simulink subsystem "In_Plane_ModelArchitecture"  (R2025b)
settings: Solver=VariableStepAuto  StartTime=0.0  StopTime=10.0  RelTol=1e-3
undefined symbols (not defined in the file or in its folder): AeroLiftCff, AeroLongDrgCff, AeroMotoEffctArea, AeroPitchMomentCff, AeroPitchMomentLngth, AeroRltWindAngVect, AeroSideFrcCff, AeroYawMomentCff, aMode, BrkFrntBrkActrBore, BrkFrntBrkActrPrsBpt, BrkFrntBrkPadMeanRadius, BrkFrntBrkTrqTbl, BrkFrntIntrnRadius, BrkFrntKinFricCff, BrkFrntPadNum, BrkFrntShoePinToDrumCntrDst, BrkFrntShoePinToFrcAppDst, BrkFrntShoePinToPadEndAng, BrkFrntShoePinToPadStartAng, BrkFrntStcFricCff, BrkFrntWhlSpdBpt, BrkRearBrkActrBore, BrkRearBrkActrPrsBpt, BrkRearBrkPadMeanRadius, BrkRearBrkTrqTbl, BrkRearIntrnRadius, BrkRearKinFricCff, BrkRearPadNum, BrkRearShoePinToDrumCntrDst, BrkRearShoePinToFrcAppDst, BrkRearShoePinToPadEndAng, BrkRearShoePinToPadStartAng, BrkRearStcFricCff, BrkRearWhlSpdBpt, EnvAbsPrs, EnvAirTemp, FrkFrL0, FrmAng0, g, GasCnst, InitFrkLngth, InitMainFrmPitchAng, InitRearArmPitchAng, InitRearCntctPtchLatVel, InitRearCntctPtchLongVel, InitRearCntctPtchY, InitRearCntctPtchZ, InitRollAng, InitYawAng, MotoFrmLngth, MotoFrmMass, MotoGrvty, MotoLatOfst, MotoLongOfst, MotoLowrFrntFrkMass, MotoPtchOfst, MotoRearArmLngth, MotoRearArmMass, MotoRollOfst ... (+25)
libraries: sm_lib x309, nesl_utility_internal x158, nesl_utility x7, autolibsharedcoupling x6, vehdynlibtire x6, sharedtransform x4, shared6dof x1, matrix_library x1, vehdynlibeomcommon x1
(part 5 of 10)

== system In_Plane_ModelArchitecture/Chassis, Tires, and Areo/Chassis Body, Suspension, and Steering/CHASSIS/Sensors/Geom sensor/Sensor_origin ==
  Demux : Demux  Outputs=3
  PS-Simulink Converter : nesl_utility_internal/PS-Simulink Converter  PhysicalDomain=network_engine_domain  SubClassName=ps_output  LeftPortType=input  RightPortType=output  PseudoPeriodic=off  Frequencies=[]  VectorFormat=1-D array  Unit=rad  AffineConversion=off
  PS-Simulink Converter1 : nesl_utility_internal/PS-Simulink Converter  PhysicalDomain=network_engine_domain  SubClassName=ps_output  LeftPortType=input  RightPortType=output  PseudoPeriodic=off  Frequencies=[]  VectorFormat=1-D array  Unit=inherit  AffineConversion=off
  PS-Simulink Converter2 : nesl_utility_internal/PS-Simulink Converter  PhysicalDomain=network_engine_domain  SubClassName=ps_output  LeftPortType=input  RightPortType=output  PseudoPeriodic=off  Frequencies=[]  VectorFormat=1-D array  Unit=inherit  AffineConversion=off
  PS-Simulink Converter3 : nesl_utility_internal/PS-Simulink Converter  PhysicalDomain=network_engine_domain  SubClassName=ps_output  LeftPortType=input  RightPortType=output  PseudoPeriodic=off  Frequencies=[]  VectorFormat=1-D array  Unit=inherit  AffineConversion=off
  SAE origin : Subsystem
  Transform Sensor : sm_lib/Frames and Transforms/Transform Sensor  MeasurementFrame=NonRotatingBase  RotationSequence=ZYX  SenseAngle=off  SenseAxis=off  SenseQ=off  SenseR=off  SenseRotationSequence=on  SenseOmegaX=off  SenseOmegaY=off  SenseOmegaZ=off  SenseOmega=off  SenseQDot=off  SenseRDot=off  SenseRotationSequenceDot=off  SenseAlphaX=off  SenseAlphaY=off  SenseAlphaZ=off  SenseAlpha=off  SenseQDDot=off  SenseRDDot=off  SenseX=on  SenseY=on  SenseZ=on  SenseXYZ=off  SenseRad=off  SenseAzim=off  SenseDist=off  SenseInc=off  SenseXDot=off  SenseYDot=off  SenseZDot=off  SenseXYZDot=off  SenseRadDot=off  SenseAzimDot=off  SenseDistDot=off  SenseIncDot=off  SenseXDDot=off  SenseYDDot=off  SenseZDDot=off  SenseXYZDDot=off  SenseRadDDot=off  SenseAzimDDot=off  SenseDistDDot=off  SenseIncDDot=off
  B : PMIOPort  Side=Left
  psi : Outport
  theta : Outport  Port=2
  phi : Outport  Port=3
  x : Outport  Port=4
  y : Outport  Port=5
  z : Outport  Port=6
  wires:
  PS-Simulink Converter3/1 -> z/1
  PS-Simulink Converter2/1 -> y/1
  PS-Simulink Converter1/1 -> x/1
  Demux/3 -> phi/1
  Demux/1 -> psi/1
  Demux/2 -> theta/1
  PS-Simulink Converter/1 -> Demux/1
  connections:
  Transform Sensor/RConn5 -- PS-Simulink Converter3/LConn1
  PS-Simulink Converter2/LConn1 -- Transform Sensor/RConn4
  PS-Simulink Converter1/LConn1 -- Transform Sensor/RConn3
  PS-Simulink Converter/LConn1 -- Transform Sensor/RConn2
  Transform Sensor/RConn1 -- B/RConn1
  Transform Sensor/LConn1 -- SAE origin/RConn1

== system In_Plane_ModelArchitecture/Chassis, Tires, and Areo/Chassis Body, Suspension, and Steering/CHASSIS/Sensors/HubFr_sensor/Origin ==
  World Frame : sm_lib/Frames and Transforms/World Frame
  X+pi : sm_lib/Frames and Transforms/Rigid Transform  RotationMethod=StandardAxis  FollAlignAxisA=+X  BaseAlignAxisA=+Y  FollAlignAxisB=+Y  BaseAlignAxisB=+Z  RotationStandardAxis=+X  RotationAngle=pi  RotationAngleUnits=rad  RotationArbitraryAxis=[0 0 1]  RotationSequenceAxes=FollowerAxes  RotationSequence=XYX  RotationSequenceAngles=[0 0 0]  RotationSequenceAnglesUnits=deg  RotationMatrix=[1 0 0; 0 1 0; 0 0 1]  Quaternion=[1 0 0 0]  TranslationMethod=None  TranslationCartesianOffset=[0 0 0]  TranslationCartesianOffsetUnits=m  TranslationStandardAxis=+Z  TranslationStandardOffset=0  TranslationStandardOffsetUnits=m  TranslationROffset=0  TranslationROffsetUnits=m  TranslationThetaOffset=0  TranslationThetaOffsetUnits=deg  TranslationZOffset=0  TranslationZOffsetUnits=m
  F : PMIOPort  Side=Right
  connections:
  World Frame/RConn1 -- X+pi/LConn1
  X+pi/RConn1 -- F/RConn1

== system In_Plane_ModelArchitecture/Chassis, Tires, and Areo/Chassis Body, Suspension, and Steering/CHASSIS/Sensors/HubFr_sensor/World vertical frame ==
  Angle Constraint : sm_lib/Constraints/Angle Constraint  ConstraintType=Parallel  Angle=pi  AngleUnits=rad  WrenchDir=FollowerOnBase  WrenchFrame=BaseFrame  SenseTorque=off  SenseSignedTorqueMagnitude=off
  Graphic1 : sm_lib/Body Elements/Graphic  GraphicType=Marker  MarkerShape=Frame  MarkerSize=40  GraphicVisPropType=SimpleVisualProperties  GraphicDiffuseColor=[1 0.07451 0.651]  GraphicOpacity=1.0  GraphicSpecularColor=[0.5 0.5 0.5 1.0]  GraphicAmbientColor=[0.15 0.15 0.15 1.0]  GraphicEmissiveColor=[0.0 0.0 0.0 1.0]  GraphicShininess=75
  Revolute Joint : sm_lib/Joints/Revolute Joint  JointMode=Normal  CompositeWrenchDir=FollowerOnBase  CompositeWrenchFrame=BaseFrame  SenseConstraintForce=off  SenseConstraintTorque=off  SenseTotalForce=off  SenseTotalTorque=off  PositionTargetSpecify=off  PositionTargetPriority=High  PositionTargetValue=0  PositionTargetValueUnits=deg  VelocityTargetSpecify=off  VelocityTargetPriority=High  VelocityTargetValue=0  VelocityTargetValueUnits=deg/s  EquilibriumPosition=0  EquilibriumPositionUnits=deg  SpringStiffness=0  SpringStiffnessUnits=N*m/deg  DampingCoefficient=0  DampingCoefficientUnits=N*m/(deg/s)  LowerLimitSpecify=off  LowerLimitBound=-90  LowerLimitBoundUnits=deg  LowerLimitStiffness=1e4  LowerLimitStiffnessUnits=N*m/deg  LowerLimitDamping=10  LowerLimitDampingUnits=N*m/(deg/s)  LowerLimitTransitionRegionWidth=0.1  LowerLimitTransitionRegionWidthUnits=deg  UpperLimitSpecify=off  UpperLimitBound=90  UpperLimitBoundUnits=deg  UpperLimitStiffness=1e4  UpperLimitStiffnessUnits=N*m/deg  UpperLimitDamping=10  UpperLimitDampingUnits=N*m/(deg/s)  UpperLimitTransitionRegionWidth=0.1  UpperLimitTransitionRegionWidthUnits=deg  TorqueActuationMode=NoTorque  MotionActuationMode=ComputedMotion  SensePosition=off  SenseVelocity=off  SenseAcceleration=off  SenseTorqueForce=off  SenseLowerLimitTorqueForce=off  SenseUpperLimitTorqueForce=off
  Revolute Joint1 : sm_lib/Joints/Revolute Joint  JointMode=Normal  CompositeWrenchDir=FollowerOnBase  CompositeWrenchFrame=BaseFrame  SenseConstraintForce=off  SenseConstraintTorque=off  SenseTotalForce=off  SenseTotalTorque=off  PositionTargetSpecify=off  PositionTargetPriority=High  PositionTargetValue=0  PositionTargetValueUnits=deg  VelocityTargetSpecify=off  VelocityTargetPriority=High  VelocityTargetValue=0  VelocityTargetValueUnits=deg/s  EquilibriumPosition=0  EquilibriumPositionUnits=deg  SpringStiffness=0  SpringStiffnessUnits=N*m/deg  DampingCoefficient=0  DampingCoefficientUnits=N*m/(deg/s)  LowerLimitSpecify=off  LowerLimitBound=-90  LowerLimitBoundUnits=deg  LowerLimitStiffness=1e4  LowerLimitStiffnessUnits=N*m/deg  LowerLimitDamping=10  LowerLimitDampingUnits=N*m/(deg/s)  LowerLimitTransitionRegionWidth=0.1  LowerLimitTransitionRegionWidthUnits=deg  UpperLimitSpecify=off  UpperLimitBound=90  UpperLimitBoundUnits=deg  UpperLimitStiffness=1e4  UpperLimitStiffnessUnits=N*m/deg  UpperLimitDamping=10  UpperLimitDampingUnits=N*m/(deg/s)  UpperLimitTransitionRegionWidth=0.1  UpperLimitTransitionRegionWidthUnits=deg  TorqueActuationMode=NoTorque  MotionActuationMode=ComputedMotion  SensePosition=off  SenseVelocity=off  SenseAcceleration=off  SenseTorqueForce=off  SenseLowerLimitTorqueForce=off  SenseUpperLimitTorqueForce=off
  Rigid Transform : sm_lib/Frames and Transforms/Rigid Transform  RotationMethod=StandardAxis  FollAlignAxisA=+X  BaseAlignAxisA=+Y  FollAlignAxisB=+Y  BaseAlignAxisB=+Z  RotationStandardAxis=+X  RotationAngle=-pi/2  RotationAngleUnits=rad  RotationArbitraryAxis=[0 0 1]  RotationSequenceAxes=FollowerAxes  RotationSequence=XYX  RotationSequenceAngles=[0 0 0]  RotationSequenceAnglesUnits=deg  RotationMatrix=[1 0 0; 0 1 0; 0 0 1]  Quaternion=[1 0 0 0]  TranslationMethod=None  TranslationCartesianOffset=[0 0 0]  TranslationCartesianOffsetUnits=m  TranslationStandardAxis=+Z  TranslationStandardOffset=0  TranslationStandardOffsetUnits=m  TranslationROffset=0  TranslationROffsetUnits=m  TranslationThetaOffset=0  TranslationThetaOffsetUnits=deg  TranslationZOffset=0  TranslationZOffsetUnits=m
  Rigid Transform1 : sm_lib/Frames and Transforms/Rigid Transform  RotationMethod=StandardAxis  FollAlignAxisA=+X  BaseAlignAxisA=+Y  FollAlignAxisB=+Y  BaseAlignAxisB=+Z  RotationStandardAxis=+Y  RotationAngle=pi/2  RotationAngleUnits=rad  RotationArbitraryAxis=[0 0 1]  RotationSequenceAxes=FollowerAxes  RotationSequence=XYX  RotationSequenceAngles=[0 0 0]  RotationSequenceAnglesUnits=deg  RotationMatrix=[1 0 0; 0 1 0; 0 0 1]  Quaternion=[1 0 0 0]  TranslationMethod=None  TranslationCartesianOffset=[0 0 0]  TranslationCartesianOffsetUnits=m  TranslationStandardAxis=+Z  TranslationStandardOffset=0  TranslationStandardOffsetUnits=m  TranslationROffset=0  TranslationROffsetUnits=m  TranslationThetaOffset=0  TranslationThetaOffsetUnits=deg  TranslationZOffset=0  TranslationZOffsetUnits=m
  Rigid Transform2 : sm_lib/Frames and Transforms/Rigid Transform  RotationMethod=StandardAxis  FollAlignAxisA=+X  BaseAlignAxisA=+Y  FollAlignAxisB=+Y  BaseAlignAxisB=+Z  RotationStandardAxis=+X  RotationAngle=pi/2  RotationAngleUnits=rad  RotationArbitraryAxis=[0 0 1]  RotationSequenceAxes=FollowerAxes  RotationSequence=XYX  RotationSequenceAngles=[0 0 0]  RotationSequenceAnglesUnits=deg  RotationMatrix=[1 0 0; 0 1 0; 0 0 1]  Quaternion=[1 0 0 0]  TranslationMethod=None  TranslationCartesianOffset=[0 0 0]  TranslationCartesianOffsetUnits=m  TranslationStandardAxis=+Z  TranslationStandardOffset=0  TranslationStandardOffsetUnits=m  TranslationROffset=0  TranslationROffsetUnits=m  TranslationThetaOffset=0  TranslationThetaOffsetUnits=deg  TranslationZOffset=0  TranslationZOffsetUnits=m
  Rigid Transform3 : sm_lib/Frames and Transforms/Rigid Transform  RotationMethod=StandardAxis  FollAlignAxisA=+X  BaseAlignAxisA=+Y  FollAlignAxisB=+Y  BaseAlignAxisB=+Z  RotationStandardAxis=+X  RotationAngle=pi  RotationAngleUnits=rad  RotationArbitraryAxis=[0 0 1]  RotationSequenceAxes=FollowerAxes  RotationSequence=XYX  RotationSequenceAngles=[0 0 0]  RotationSequenceAnglesUnits=deg  RotationMatrix=[1 0 0; 0 1 0; 0 0 1]  Quaternion=[1 0 0 0]  TranslationMethod=None  TranslationCartesianOffset=[0 0 0]  TranslationCartesianOffsetUnits=m  TranslationStandardAxis=+X  TranslationStandardOffset=0  TranslationStandardOffsetUnits=m  TranslationROffset=0  TranslationROffsetUnits=m  TranslationThetaOffset=0  TranslationThetaOffsetUnits=deg  TranslationZOffset=0  TranslationZOffsetUnits=m
  Rigid Transform4 : sm_lib/Frames and Transforms/Rigid Transform  RotationMethod=StandardAxis  FollAlignAxisA=+X  BaseAlignAxisA=+Y  FollAlignAxisB=+Y  BaseAlignAxisB=+Z  RotationStandardAxis=+Z  RotationAngle=pi/2  RotationAngleUnits=rad  RotationArbitraryAxis=[0 0 1]  RotationSequenceAxes=FollowerAxes  RotationSequence=XYX  RotationSequenceAngles=[0 0 0]  RotationSequenceAnglesUnits=deg  RotationMatrix=[1 0 0; 0 1 0; 0 0 1]  Quaternion=[1 0 0 0]  TranslationMethod=None  TranslationCartesianOffset=[0 0 0]  TranslationCartesianOffsetUnits=m  TranslationStandardAxis=+Z  TranslationStandardOffset=0  TranslationStandardOffsetUnits=m  TranslationROffset=0  TranslationROffsetUnits=m  TranslationThetaOffset=0  TranslationThetaOffsetUnits=deg  TranslationZOffset=0  TranslationZOffsetUnits=m
  Spherical Solid : sm_lib/Body Elements/Spherical Solid  SphereRadius=0.001  SphereRadiusUnits=m  ExportEntireGeometry=off  InertiaType=Custom  BasedOnType=Density  Density=1000  DensityUnits=kg/m^3  Mass=1e-3  MassUnits=kg  CenterOfMass=[0 0 0]  CenterOfMassUnits=m  MomentsOfInertia=[1 1 1]*1e-6  MomentsOfInertiaUnits=kg*m^2  ProductsOfInertia=[0 0 0]  ProductsOfInertiaUnits=kg*m^2  GraphicType=FromGeometry  MarkerShape=Sphere  MarkerSize=10  GraphicVisPropType=SimpleVisualProperties  GraphicDiffuseColor=[0.5 0.5 0.5]  GraphicOpacity=1.0  GraphicSpecularColor=[0.5 0.5 0.5 1.0]  GraphicAmbientColor=[0.15 0.15 0.15 1.0]  GraphicEmissiveColor=[0.0 0.0 0.0 1.0]  GraphicShininess=75  DoExposeReferenceFrame=on  SerializedFrames=<Frames/>
  World Frame : sm_lib/Frames and Transforms/World Frame
  B : PMIOPort  Side=Left
  F : PMIOPort  Port=2  Side=Right
  connections:
  Rigid Transform4/LConn1 -- Rigid Transform2/RConn1
  Rigid Transform1/LConn1 -- Revolute Joint/RConn1
  Graphic1/RConn1 -- Angle Constraint/LConn1 -- Rigid Transform4/RConn1 -- F/RConn1 -- Spherical Solid/RConn1
  Revolute Joint/LConn1 -- Rigid Transform/RConn1
  Revolute Joint1/LConn1 -- Rigid Transform1/RConn1
  Rigid Transform2/LConn1 -- Revolute Joint1/RConn1
  Rigid Transform3/LConn1 -- World Frame/RConn1
  Angle Constraint/RConn1 -- Rigid Transform3/RConn1
  Rigid Transform/LConn1 -- B/RConn1

== system In_Plane_ModelArchitecture/Chassis, Tires, and Areo/Chassis Body, Suspension, and Steering/CHASSIS/Steering and fork/Fork/fork (dofPrism) ==
  f : Inport
  Bus Creator : BusCreator  Inputs=3
  Selector2 : Selector  InputPortWidth=3  IndexOptions=Index vector (dialog)  Indices=3  OutputSizes=1
  fork : Subsystem  Variant=on  VariantControlMode=label  VariantControl=Choice  LabelModeActiveChoice=fork
  B : PMIOPort  Side=Left
  F : PMIOPort  Port=2  Side=Right
  Lfrk : Outport
  FrkFz : Outport  Port=2
  wires:
  f/1 -> fork/1(f)
  Selector2/1 -> FrkFz/1
  Bus Creator/1 -> Lfrk/1  "Lfrk"
  fork/4(ft) -> Selector2/1  "ft"
  fork/3(a) -> Bus Creator/1  "LfrkA"
  fork/2(v) -> Bus Creator/2  "LfrkV"
  fork/1(p) -> Bus Creator/3  "LfrkPz"
  connections:
  fork/RConn1 -- F/RConn1
  fork/LConn1 -- B/RConn1

== system In_Plane_ModelArchitecture/Chassis, Tires, and Areo/Chassis Body, Suspension, and Steering/CHASSIS/Steering and fork/Fork/mass_FrkLw ==
  CG_Solid : sm_lib/Body Elements/Spherical Solid  SphereRadius=3e-2  SphereRadiusUnits=m  ExportEntireGeometry=off  InertiaType=Custom  BasedOnType=Density  Density=1000  DensityUnits=kg/m^3  Mass=MotoLowrFrntFrkMass  MassUnits=kg  CenterOfMass=[0 0 0]  CenterOfMassUnits=m  MomentsOfInertia=MotoLowrFrntFrkInert  MomentsOfInertiaUnits=kg*m^2  ProductsOfInertia=[0 0 0]  ProductsOfInertiaUnits=kg*m^2  GraphicType=FromGeometry  MarkerShape=Sphere  MarkerSize=10  GraphicVisPropType=SimpleVisualProperties  GraphicDiffuseColor=[1.0 0.0 0.0]  GraphicOpacity=1.0  GraphicSpecularColor=[0.5 0.5 0.5 1.0]  GraphicAmbientColor=[0.15 0.15 0.15 1.0]  GraphicEmissiveColor=[0.0 0.0 0.0 1.0]  GraphicShininess=75  DoExposeReferenceFrame=on  SerializedFrames=<Frames/>
  CofGCoord. : sm_lib/Frames and Transforms/Rigid Transform  RotationMethod=None  FollAlignAxisA=+X  BaseAlignAxisA=+Y  FollAlignAxisB=+Y  BaseAlignAxisB=+Z  RotationStandardAxis=+X  RotationAngle=0  RotationAngleUnits=rad  RotationArbitraryAxis=[0 0 1]  RotationSequenceAxes=FollowerAxes  RotationSequence=XYX  RotationSequenceAngles=[0 0 0]  RotationSequenceAnglesUnits=deg  RotationMatrix=[1 0 0; 0 1 0; 0 0 1]  Quaternion=[1 0 0 0]  TranslationMethod=Cartesian  TranslationCartesianOffset=MotoLowrFrntFrkPos  TranslationCartesianOffsetUnits=m  TranslationStandardAxis=+X  TranslationStandardOffset=0  TranslationStandardOffsetUnits=m  TranslationROffset=0  TranslationROffsetUnits=m  TranslationThetaOffset=0  TranslationThetaOffsetUnits=deg  TranslationZOffset=0  TranslationZOffsetUnits=m
  Graphic : sm_lib/Body Elements/Graphic  GraphicType=Marker  MarkerShape=Frame  MarkerSize=30  GraphicVisPropType=SimpleVisualProperties  GraphicDiffuseColor=[0.0 0.0 1.0]  GraphicOpacity=1.0  GraphicSpecularColor=[0.5 0.5 0.5 1.0]  GraphicAmbientColor=[0.15 0.15 0.15 1.0]  GraphicEmissiveColor=[0.0 0.0 0.0 1.0]  GraphicShininess=75
  World vertical frame : Subsystem  VariantControl=World vertical
  B : PMIOPort  Side=Left
  CG : PMIOPort  Port=2  Side=Right
  WVFrame_FrkLw : PMIOPort  Port=3  Side=Right
  connections:
  World vertical frame/RConn1 -- WVFrame_FrkLw/RConn1
  CofGCoord./LConn1 -- B/RConn1 -- Graphic/RConn1
  CofGCoord./RConn1 -- CG/RConn1 -- World vertical frame/LConn1 -- CG_Solid/RConn1

== system In_Plane_ModelArchitecture/Chassis, Tires, and Areo/Chassis Body, Suspension, and Steering/CHASSIS/Steering and fork/Fork/mass_FrkUp ==
  CGCoord. : sm_lib/Frames and Transforms/Rigid Transform  RotationMethod=None  FollAlignAxisA=+X  BaseAlignAxisA=+Y  FollAlignAxisB=+Y  BaseAlignAxisB=+Z  RotationStandardAxis=+X  RotationAngle=0  RotationAngleUnits=rad  RotationArbitraryAxis=[0 0 1]  RotationSequenceAxes=FollowerAxes  RotationSequence=XYX  RotationSequenceAngles=[0 0 0]  RotationSequenceAnglesUnits=deg  RotationMatrix=[1 0 0; 0 1 0; 0 0 1]  Quaternion=[1 0 0 0]  TranslationMethod=Cartesian  TranslationCartesianOffset=MotoUpprFrntFrkPos  TranslationCartesianOffsetUnits=m  TranslationStandardAxis=+X  TranslationStandardOffset=0  TranslationStandardOffsetUnits=m  TranslationROffset=0  TranslationROffsetUnits=m  TranslationThetaOffset=0  TranslationThetaOffsetUnits=deg  TranslationZOffset=0  TranslationZOffsetUnits=m
  CG_Solid : sm_lib/Body Elements/Spherical Solid  SphereRadius=3e-2  SphereRadiusUnits=m  ExportEntireGeometry=off  InertiaType=Custom  BasedOnType=Density  Density=1000  DensityUnits=kg/m^3  Mass=MotoUpprFrntFrkMass  MassUnits=kg  CenterOfMass=[0 0 0]  CenterOfMassUnits=m  MomentsOfInertia=MotoUpprFrntFrkInert  MomentsOfInertiaUnits=kg*m^2  ProductsOfInertia=[0 0 0]  ProductsOfInertiaUnits=kg*m^2  GraphicType=FromGeometry  MarkerShape=Sphere  MarkerSize=10  GraphicVisPropType=SimpleVisualProperties  GraphicDiffuseColor=[1.0 0.0 0.0]  GraphicOpacity=1.0  GraphicSpecularColor=[0.5 0.5 0.5 1.0]  GraphicAmbientColor=[0.15 0.15 0.15 1.0]  GraphicEmissiveColor=[0.0 0.0 0.0 1.0]  GraphicShininess=75  DoExposeReferenceFrame=on  SerializedFrames=<Frames/>
  Graphic : sm_lib/Body Elements/Graphic  GraphicType=Marker  MarkerShape=Frame  MarkerSize=30  GraphicVisPropType=SimpleVisualProperties  GraphicDiffuseColor=[0.0 0.0 1.0]  GraphicOpacity=1.0  GraphicSpecularColor=[0.5 0.5 0.5 1.0]  GraphicAmbientColor=[0.15 0.15 0.15 1.0]  GraphicEmissiveColor=[0.0 0.0 0.0 1.0]  GraphicShininess=75
  World vertical frame : Subsystem  VariantControl=World vertical
  B : PMIOPort  Side=Left
  WVFrame_FrkUp : PMIOPort  Port=2  Side=Right
  connections:
  World vertical frame/RConn1 -- WVFrame_FrkUp/RConn1
  World vertical frame/LConn1 -- CGCoord./RConn1 -- CG_Solid/RConn1
  CGCoord./LConn1 -- B/RConn1 -- Graphic/RConn1

== system In_Plane_ModelArchitecture/Chassis, Tires, and Areo/Chassis Body, Suspension, and Steering/CHASSIS/Steering and fork/Fork/offset ==
  Graphic : sm_lib/Body Elements/Graphic  GraphicType=Marker  MarkerShape=Frame  MarkerSize=30  GraphicVisPropType=SimpleVisualProperties  GraphicDiffuseColor=[0.0 0.0 1.0]  GraphicOpacity=1.0  GraphicSpecularColor=[0.5 0.5 0.5 1.0]  GraphicAmbientColor=[0.15 0.15 0.15 1.0]  GraphicEmissiveColor=[0.0 0.0 0.0 1.0]  GraphicShininess=75
  offset : sm_lib/Frames and Transforms/Rigid Transform  RotationMethod=None  FollAlignAxisA=+X  BaseAlignAxisA=+Y  FollAlignAxisB=+Y  BaseAlignAxisB=+Z  RotationStandardAxis=+X  RotationAngle=0  RotationAngleUnits=rad  RotationArbitraryAxis=[0 0 1]  RotationSequenceAxes=FollowerAxes  RotationSequence=XYX  RotationSequenceAngles=[0 0 0]  RotationSequenceAnglesUnits=deg  RotationMatrix=[1 0 0; 0 1 0; 0 0 1]  Quaternion=[1 0 0 0]  TranslationMethod=Cartesian  TranslationCartesianOffset=[MotoUpprFrntFrkOfst 0 0]  TranslationCartesianOffsetUnits=m  TranslationStandardAxis=+X  TranslationStandardOffset=0  TranslationStandardOffsetUnits=m  TranslationROffset=0  TranslationROffsetUnits=m  TranslationThetaOffset=0  TranslationThetaOffsetUnits=deg  TranslationZOffset=0  TranslationZOffsetUnits=m
  B : PMIOPort  Side=Left
  F : PMIOPort  Port=2  Side=Right
  connections:
  Graphic/RConn1 -- offset/RConn1 -- F/RConn1
  offset/LConn1 -- B/RConn1

== system In_Plane_ModelArchitecture/Chassis, Tires, and Areo/Chassis Body, Suspension, and Steering/CHASSIS/Steering and fork/Steering/Steering damper ==
  StrAngV : Inport
  MStrDmpin : Inport  Port=2
  No_Damper : Subsystem  VariantControl=No_Damper  ReferencedSubsystem=No_Damper
  MStrDmp : Outport

== system In_Plane_ModelArchitecture/Chassis, Tires, and Areo/Chassis Body, Suspension, and Steering/CHASSIS/Steering and fork/Steering/Str dof ==
  t : Inport
  No_Steering : Subsystem  VariantControl=No_Steering  ReferencedSubsystem=No_Steering
  B : PMIOPort  Side=Left
  F : PMIOPort  Port=2  Side=Right
  b : Outport
  w : Outport  Port=2
  q : Outport  Port=3

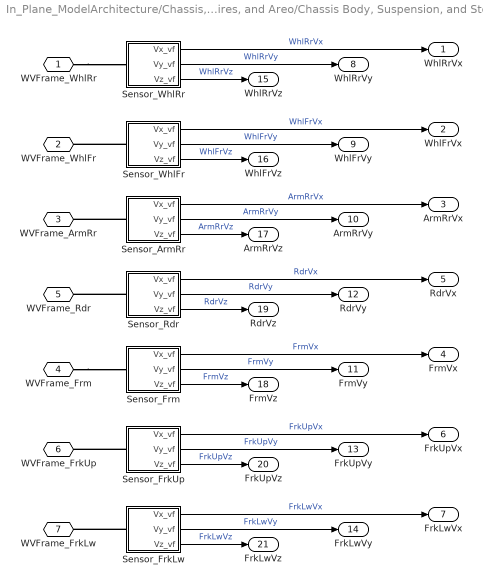
== system In_Plane_ModelArchitecture/Chassis, Tires, and Areo/Chassis Body, Suspension, and Steering/Signal routine/Ancillary_sub/Velocities/Sensor ==
  Sensor_ArmRr : Subsystem
  Sensor_FrkLw : Subsystem
  Sensor_FrkUp : Subsystem
  Sensor_Frm : Subsystem
  Sensor_Rdr : Subsystem
  Sensor_WhlFr : Subsystem
  Sensor_WhlRr : Subsystem
  WVFrame_WhlRr : PMIOPort  Side=Left
  WVFrame_WhlFr : PMIOPort  Port=2  Side=Left
  WVFrame_ArmRr : PMIOPort  Port=3  Side=Left
  WVFrame_Frm : PMIOPort  Port=4  Side=Left
  WVFrame_Rdr : PMIOPort  Port=5  Side=Left
  WVFrame_FrkUp : PMIOPort  Port=6  Side=Left
  WVFrame_FrkLw : PMIOPort  Port=7  Side=Left
  WhlRrVx : Outport
  WhlFrVx : Outport  Port=2
  ArmRrVx : Outport  Port=3
  FrmVx : Outport  Port=4
  RdrVx : Outport  Port=5
  FrkUpVx : Outport  Port=6
  FrkLwVx : Outport  Port=7
  WhlRrVy : Outport  Port=8
  WhlFrVy : Outport  Port=9
  ArmRrVy : Outport  Port=10
  FrmVy : Outport  Port=11
  RdrVy : Outport  Port=12
  FrkUpVy : Outport  Port=13
  FrkLwVy : Outport  Port=14
  WhlRrVz : Outport  Port=15
  WhlFrVz : Outport  Port=16
  ArmRrVz : Outport  Port=17
  FrmVz : Outport  Port=18
  RdrVz : Outport  Port=19
  FrkUpVz : Outport  Port=20
  FrkLwVz : Outport  Port=21
  wires:
  Sensor_Rdr/3(Vz_vf) -> RdrVz/1  "RdrVz"
  Sensor_Rdr/1(Vx_vf) -> RdrVx/1  "RdrVx"
  Sensor_Rdr/2(Vy_vf) -> RdrVy/1  "RdrVy"
  Sensor_FrkLw/1(Vx_vf) -> FrkLwVx/1  "FrkLwVx"
  Sensor_WhlRr/2(Vy_vf) -> WhlRrVy/1  "WhlRrVy"
  Sensor_ArmRr/2(Vy_vf) -> ArmRrVy/1  "ArmRrVy"
  Sensor_FrkUp/2(Vy_vf) -> FrkUpVy/1  "FrkUpVy"
  Sensor_ArmRr/3(Vz_vf) -> ArmRrVz/1  "ArmRrVz"
  Sensor_WhlFr/1(Vx_vf) -> WhlFrVx/1  "WhlFrVx"
  Sensor_WhlFr/3(Vz_vf) -> WhlFrVz/1  "WhlFrVz"
  Sensor_FrkUp/3(Vz_vf) -> FrkUpVz/1  "FrkUpVz"
  Sensor_FrkLw/2(Vy_vf) -> FrkLwVy/1  "FrkLwVy"
  Sensor_ArmRr/1(Vx_vf) -> ArmRrVx/1  "ArmRrVx"
  Sensor_FrkUp/1(Vx_vf) -> FrkUpVx/1  "FrkUpVx"
  Sensor_Frm/1(Vx_vf) -> FrmVx/1  "FrmVx"
  Sensor_Frm/2(Vy_vf) -> FrmVy/1  "FrmVy"
  Sensor_WhlRr/3(Vz_vf) -> WhlRrVz/1  "WhlRrVz"
  Sensor_Frm/3(Vz_vf) -> FrmVz/1  "FrmVz"
  Sensor_WhlFr/2(Vy_vf) -> WhlFrVy/1  "WhlFrVy"
  Sensor_FrkLw/3(Vz_vf) -> FrkLwVz/1  "FrkLwVz"
  Sensor_WhlRr/1(Vx_vf) -> WhlRrVx/1  "WhlRrVx"
  connections:
  Sensor_Rdr/LConn1 -- WVFrame_Rdr/RConn1
  Sensor_WhlFr/LConn1 -- WVFrame_WhlFr/RConn1
  WVFrame_WhlRr/RConn1 -- Sensor_WhlRr/LConn1
  Sensor_FrkLw/LConn1 -- WVFrame_FrkLw/RConn1
  WVFrame_Frm/RConn1 -- Sensor_Frm/LConn1
  Sensor_ArmRr/LConn1 -- WVFrame_ArmRr/RConn1
  Sensor_FrkUp/LConn1 -- WVFrame_FrkUp/RConn1

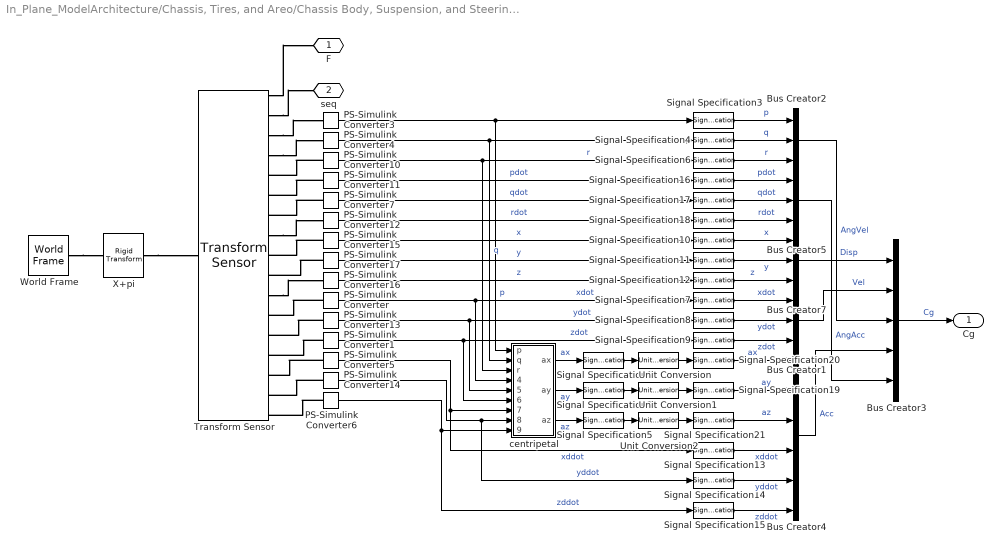
== system In_Plane_ModelArchitecture/Chassis, Tires, and Areo/Chassis Body, Suspension, and Steering/Signal routine/Info_sub/BdyFrm/CG ==
  Bus Creator{1..2,5,7} (4 alike) : BusCreator  Inputs=3
  Bus Creator3 : BusCreator  Inputs=5
  Bus Creator4 : BusCreator  Inputs=6
  PS-Simulink Converter{,1,3..7,10..17} (15 alike) : nesl_utility_internal/PS-Simulink Converter  PhysicalDomain=network_engine_domain  SubClassName=ps_output  LeftPortType=input  RightPortType=output  PseudoPeriodic=off  Frequencies=[]  VectorFormat=1-D array  Unit=inherit  AffineConversion=off
  Signal Specification{1..2,5,13..15} (6 alike) : SignalSpecification  Unit=m/s^2
  Signal Specification10 : SignalSpecification  Unit=m
  Signal Specification11 : SignalSpecification  Unit=m
  Signal Specification12 : SignalSpecification  Unit=m
  Signal Specification16 : SignalSpecification  Unit=rad/s^2
  Signal Specification17 : SignalSpecification  Unit=rad/s^2
  Signal Specification18 : SignalSpecification  Unit=rad/s^2
  Signal Specification19 : SignalSpecification  Unit=gn
  Signal Specification20 : SignalSpecification  Unit=gn
  Signal Specification21 : SignalSpecification  Unit=gn
  Signal Specification3 : SignalSpecification  Unit=rad/s
  Signal Specification4 : SignalSpecification  Unit=rad/s
  Signal Specification6 : SignalSpecification  Unit=rad/s
  Signal Specification7 : SignalSpecification  Unit=m/s
  Signal Specification8 : SignalSpecification  Unit=m/s
  Signal Specification9 : SignalSpecification  Unit=m/s
  Transform Sensor : sm_lib/Frames and Transforms/Transform Sensor  MeasurementFrame=NonRotatingFollower  RotationSequence=ZYX  SenseAngle=off  SenseAxis=off  SenseQ=off  SenseR=off  SenseRotationSequence=on  SenseOmegaX=on  SenseOmegaY=on  SenseOmegaZ=on  SenseOmega=off  SenseQDot=off  SenseRDot=off  SenseRotationSequenceDot=off  SenseAlphaX=on  SenseAlphaY=on  SenseAlphaZ=on  SenseAlpha=off  SenseQDDot=off  SenseRDDot=off  SenseX=on  SenseY=on  SenseZ=on  SenseXYZ=off  SenseRad=off  SenseAzim=off  SenseDist=off  SenseInc=off  SenseXDot=on  SenseYDot=on  SenseZDot=on  SenseXYZDot=off  SenseRadDot=off  SenseAzimDot=off  SenseDistDot=off  SenseIncDot=off  SenseXDDot=on  SenseYDDot=on  SenseZDDot=on  SenseXYZDDot=off  SenseRadDDot=off  SenseAzimDDot=off  SenseDistDDot=off  SenseIncDDot=off
  Unit Conversion : UnitConversion
  Unit Conversion1 : UnitConversion
  Unit Conversion2 : UnitConversion
  World Frame : sm_lib/Frames and Transforms/World Frame
  X+pi : sm_lib/Frames and Transforms/Rigid Transform  RotationMethod=StandardAxis  FollAlignAxisA=+X  BaseAlignAxisA=+Y  FollAlignAxisB=+Y  BaseAlignAxisB=+Z  RotationStandardAxis=+X  RotationAngle=pi  RotationAngleUnits=rad  RotationArbitraryAxis=[0 0 1]  RotationSequenceAxes=FollowerAxes  RotationSequence=XYX  RotationSequenceAngles=[0 0 0]  RotationSequenceAnglesUnits=deg  RotationMatrix=[1 0 0; 0 1 0; 0 0 1]  Quaternion=[1 0 0 0]  TranslationMethod=None  TranslationCartesianOffset=[0 0 0]  TranslationCartesianOffsetUnits=m  TranslationStandardAxis=+Z  TranslationStandardOffset=0  TranslationStandardOffsetUnits=m  TranslationROffset=0  TranslationROffsetUnits=m  TranslationThetaOffset=0  TranslationThetaOffsetUnits=deg  TranslationZOffset=0  TranslationZOffsetUnits=m
  centripetal : Subsystem
  F : PMIOPort  Side=Left
  seq : PMIOPort  Port=2  Side=Left
  Cg : Outport
  wires:
  centripetal/3(az) -> Signal Specification5/1  "az"
  centripetal/2(ay) -> Signal Specification2/1  "ay"
  centripetal/1(ax) -> Signal Specification1/1  "ax"
  Unit Conversion/1 -> Signal Specification20/1
  Unit Conversion1/1 -> Signal Specification19/1
  Unit Conversion2/1 -> Signal Specification21/1
  Signal Specification1/1 -> Unit Conversion/1
  Signal Specification2/1 -> Unit Conversion1/1
  Signal Specification5/1 -> Unit Conversion2/1
  PS-Simulink Converter1/1 -> Signal Specification9/1, centripetal/6(zdot)  "zdot"
  PS-Simulink Converter13/1 -> centripetal/5(ydot), Signal Specification8/1  "ydot"
  Bus Creator1/1 -> Bus Creator3/2  "Vel"
  PS-Simulink Converter4/1 -> centripetal/2(q), Signal Specification4/1  "q"
  PS-Simulink Converter3/1 -> centripetal/1(p), Signal Specification3/1  "p"
  PS-Simulink Converter10/1 -> centripetal/3(r), Signal Specification6/1  "r"
  Bus Creator2/1 -> Bus Creator3/3  "AngVel"
  PS-Simulink Converter5/1 -> Signal Specification13/1, centripetal/7(xddot)  "xddot"
  Bus Creator4/1 -> Bus Creator3/4  "Acc"
  Bus Creator5/1 -> Bus Creator3/5  "AngAcc"
  PS-Simulink Converter12/1 -> Signal Specification18/1  "rdot"
  PS-Simulink Converter11/1 -> Signal Specification16/1  "pdot"
  PS-Simulink Converter7/1 -> Signal Specification17/1  "qdot"
  Bus Creator3/1 -> Cg/1  "Cg"
  PS-Simulink Converter14/1 -> Signal Specification14/1, centripetal/8(yddot)  "yddot"
  PS-Simulink Converter/1 -> Signal Specification7/1, centripetal/4(xdot)  "xdot"
  PS-Simulink Converter6/1 -> Signal Specification15/1, centripetal/9(zddot)  "zddot"
  Signal Specification3/1 -> Bus Creator2/1  "p"
  Signal Specification4/1 -> Bus Creator2/2  "q"
  Signal Specification6/1 -> Bus Creator2/3  "r"
  Signal Specification7/1 -> Bus Creator1/1  "xdot"
  Signal Specification8/1 -> Bus Creator1/2  "ydot"
  Signal Specification9/1 -> Bus Creator1/3  "zdot"
  Signal Specification13/1 -> Bus Creator4/4  "xddot"
  Signal Specification14/1 -> Bus Creator4/5  "yddot"
  Signal Specification16/1 -> Bus Creator5/1  "pdot"
  Signal Specification17/1 -> Bus Creator5/2  "qdot"
  Signal Specification18/1 -> Bus Creator5/3  "rdot"
  Signal Specification19/1 -> Bus Creator4/2  "ay"
  Signal Specification21/1 -> Bus Creator4/3  "az"
  Signal Specification20/1 -> Bus Creator4/1  "ax"
  Signal Specification15/1 -> Bus Creator4/6  "zddot"
  PS-Simulink Converter15/1 -> Signal Specification10/1  "x"
  PS-Simulink Converter17/1 -> Signal Specification11/1  "y"
  PS-Simulink Converter16/1 -> Signal Specification12/1  "z"
  Signal Specification10/1 -> Bus Creator7/1  "x"
  Signal Specification11/1 -> Bus Creator7/2  "y"
  Signal Specification12/1 -> Bus Creator7/3  "z"
  Bus Creator7/1 -> Bus Creator3/1  "Disp"
  connections:
  X+pi/RConn1 -- Transform Sensor/LConn1
  Transform Sensor/RConn1 -- F/RConn1
  Transform Sensor/RConn4 -- PS-Simulink Converter4/LConn1
  PS-Simulink Converter7/LConn1 -- Transform Sensor/RConn7
  PS-Simulink Converter/LConn1 -- Transform Sensor/RConn12
  PS-Simulink Converter1/LConn1 -- Transform Sensor/RConn14
  PS-Simulink Converter5/LConn1 -- Transform Sensor/RConn15
  PS-Simulink Converter6/LConn1 -- Transform Sensor/RConn17
  Transform Sensor/RConn3 -- PS-Simulink Converter3/LConn1
  PS-Simulink Converter10/LConn1 -- Transform Sensor/RConn5
  PS-Simulink Converter11/LConn1 -- Transform Sensor/RConn6
  Transform Sensor/RConn8 -- PS-Simulink Converter12/LConn1
  PS-Simulink Converter13/LConn1 -- Transform Sensor/RConn13
  PS-Simulink Converter14/LConn1 -- Transform Sensor/RConn16
  PS-Simulink Converter15/LConn1 -- Transform Sensor/RConn9
  PS-Simulink Converter17/LConn1 -- Transform Sensor/RConn10
  Transform Sensor/RConn11 -- PS-Simulink Converter16/LConn1
  Transform Sensor/RConn2 -- seq/RConn1
  World Frame/RConn1 -- X+pi/LConn1

== system In_Plane_ModelArchitecture/Chassis, Tires, and Areo/Chassis Body, Suspension, and Steering/Signal routine/Info_sub/BdyFrm/Forces ==
  Fext_BF : Inport
  Fg : Inport  Port=2
  Fd : Inport  Port=3
  Bus Creator{3,17,20,23} (4 alike) : BusCreator  Inputs=3
  Demux : Demux  Outputs=3
  Demux1 : Demux  Outputs=3
  Demux2 : Demux  Outputs=3
  Signal Specification{1,8,14..19,25} (9 alike) : SignalSpecification  Unit=N
  Forces : Outport
  wires:
  Demux1/3 -> Signal Specification25/1
  Demux1/1 -> Signal Specification1/1
  Signal Specification18/1 -> Bus Creator17/2  "Fy"
  Bus Creator23/1 -> Bus Creator20/3  "Grvty"
  Bus Creator17/1 -> Bus Creator20/2  "Drag"
  Signal Specification14/1 -> Bus Creator23/1  "Fx"
  Demux2/1 -> Signal Specification14/1
  Signal Specification8/1 -> Bus Creator3/2  "Fy"
  Demux1/2 -> Signal Specification8/1
  Signal Specification16/1 -> Bus Creator23/3  "Fz"
  Signal Specification15/1 -> Bus Creator23/2  "Fy"
  Signal Specification1/1 -> Bus Creator3/1  "Fx"
  Signal Specification25/1 -> Bus Creator3/3  "Fz"
  Demux2/3 -> Signal Specification16/1
  Signal Specification19/1 -> Bus Creator17/3  "Fz"
  Demux/2 -> Signal Specification18/1
  Signal Specification17/1 -> Bus Creator17/1  "Fx"
  Demux/3 -> Signal Specification19/1
  Bus Creator3/1 -> Bus Creator20/1  "Ext"
  Demux/1 -> Signal Specification17/1
  Demux2/2 -> Signal Specification15/1
  Bus Creator20/1 -> Forces/1  "Forces"
  Fd/1 -> Demux/1
  Fext_BF/1 -> Demux1/1
  Fg/1 -> Demux2/1

== system In_Plane_ModelArchitecture/Chassis, Tires, and Areo/Chassis Body, Suspension, and Steering/Signal routine/Info_sub/BdyFrm/Moments ==
  Mext : Inport
  Md : Inport  Port=2
  Bus Creator1 : BusCreator  Inputs=3
  Bus Creator3 : BusCreator  Inputs=3
  Bus Creator7 : BusCreator  Inputs=2
  Demux : Demux  Outputs=3
  Demux4 : Demux  Outputs=3
  Signal Specification{3..8} (6 alike) : SignalSpecification  Unit=N*m
  Moments : Outport
  wires:
  Signal Specification4/1 -> Bus Creator1/3  "Mz"
  Bus Creator1/1 -> Bus Creator7/1  "Drag"
  Demux4/1 -> Signal Specification5/1
  Signal Specification7/1 -> Bus Creator3/3  "Mz"
  Signal Specification5/1 -> Bus Creator1/1  "Mx"
  Signal Specification3/1 -> Bus Creator1/2  "My"
  Signal Specification6/1 -> Bus Creator3/2  "My"
  Bus Creator3/1 -> Bus Creator7/2  "Ext"
  Signal Specification8/1 -> Bus Creator3/1  "Mx"
  Demux4/3 -> Signal Specification4/1
  Demux4/2 -> Signal Specification3/1
  Bus Creator7/1 -> Moments/1  "Moments"
  Md/1 -> Demux4/1
  Demux/3 -> Signal Specification7/1
  Demux/1 -> Signal Specification8/1
  Demux/2 -> Signal Specification6/1
  Mext/1 -> Demux/1

== system In_Plane_ModelArchitecture/Chassis, Tires, and Areo/Chassis Body, Suspension, and Steering/Signal routine/Info_sub/InertFrm/Convert to +Z down ==
  seq : Inport
  X : Inport  Port=2
  Y : Inport  Port=3
  Z : Inport  Port=4
  Xdot : Inport  Port=5
  Ydot : Inport  Port=6
  Zdot : Inport  Port=7
  Angle Wrap : vehdynlibeomcommon/6 DOF Generic Vehicle Body/SignalCollection/Angle Wrap  SystemSampleTime=-1  VariantControl=Variant1  LabelModeActiveChoice=Unwrap  VariantActivationTime=update diagram  EmptyChoice=off  PassThrough=off  PassThroughVariantControl=(default)  EmptyChoiceVariantControl=(default)  AllowFlexibleInterface=on  Latency=0  AutoFrameSizeCalculation=off
      link override Unwrap/Unwrap: aMode=6
  Bus Creator{,1..3} (4 alike) : BusCreator  Inputs=3
  Constant : Constant  Value=[0i;0;0]  SampleTime=-1
  Demux1 : Demux  Outputs=3
  Demux2 : Demux  Outputs=3
  Demux3 : Demux  Outputs=3
  Divide1 : Product  Inputs=**  Multiplication=Matrix(*)
  Divide2 : Product  Inputs=**  Multiplication=Matrix(*)
  Divide3 : Product  Inputs=**  Multiplication=Matrix(*)
  Matrix Concatenate : Concatenate  NumInputs=1  Mode=Multidimensional array
  Matrix Concatenate1 : Concatenate  NumInputs=3  Mode=Multidimensional array
  Matrix Concatenate2 : Concatenate  NumInputs=3  Mode=Multidimensional array
  Rotation Angles to Direction Cosine Matrix : sharedtransform/Rotation Angles to Direction Cosine Matrix  rotationOrder=ZYX  aMode=2
  Rotation Angles to Direction Cosine Matrix1 : sharedtransform/Rotation Angles to Direction Cosine Matrix  rotationOrder=ZYX  aMode=2
  Rotation Angles to Direction Cosine Matrix2 : sharedtransform/Rotation Angles to Direction Cosine Matrix  rotationOrder=ZYX  aMode=2
  Selector{,1..3} (4 alike) : Selector  InputPortWidth=3  IndexOptions=Index vector (dialog)  Indices=[3 2 1]  OutputSizes=1
  Signal Specification10 : SignalSpecification  Unit=m/s
  Signal Specification11 : SignalSpecification  Unit=rad
  Signal Specification12 : SignalSpecification  Unit=m
  Cg : Outport
  wires:
  Bus Creator1/1 -> Bus Creator/3  "Ang"
  Bus Creator2/1 -> Bus Creator/1  "Disp"
  Bus Creator3/1 -> Bus Creator/2  "Vel"
  Selector3/1 -> Matrix Concatenate/1
  seq/1 -> Selector3/1
  Signal Specification11/1 -> Demux1/1
  Demux1/1 -> Bus Creator1/1  "phi"
  Demux1/2 -> Bus Creator1/2  "theta"
  Angle Wrap/1 -> Signal Specification11/1
  Matrix Concatenate/1 -> Divide1/2
  Divide1/1 -> Angle Wrap/1
  Selector/1 -> Rotation Angles to Direction Cosine Matrix/1
  Rotation Angles to Direction Cosine Matrix/1 -> Divide1/1
  Demux2/2 -> Bus Creator2/2  "Y"
  Demux3/3 -> Bus Creator3/3  "Zdot"
  Demux2/3 -> Bus Creator2/3  "Z"
  Demux3/2 -> Bus Creator3/2  "Ydot"
  Demux3/1 -> Bus Creator3/1  "Xdot"
  Demux2/1 -> Bus Creator2/1  "X"
  Demux1/3 -> Bus Creator1/3  "psi"
  Matrix Concatenate1/1 -> Divide2/2
  X/1 -> Matrix Concatenate1/1
  Rotation Angles to Direction Cosine Matrix1/1 -> Divide2/1
  Selector1/1 -> Rotation Angles to Direction Cosine Matrix1/1
  Divide2/1 -> Signal Specification12/1
  Y/1 -> Matrix Concatenate1/2
  Z/1 -> Matrix Concatenate1/3
  Zdot/1 -> Matrix Concatenate2/3
  Ydot/1 -> Matrix Concatenate2/2
  Selector2/1 -> Rotation Angles to Direction Cosine Matrix2/1
  Rotation Angles to Direction Cosine Matrix2/1 -> Divide3/1
  Constant/1 -> Selector1/1, Selector2/1, Selector/1
  Xdot/1 -> Matrix Concatenate2/1
  Matrix Concatenate2/1 -> Divide3/2
  Divide3/1 -> Signal Specification10/1
  Bus Creator/1 -> Cg/1
  Signal Specification10/1 -> Demux3/1
  Signal Specification12/1 -> Demux2/1

== system In_Plane_ModelArchitecture/Chassis, Tires, and Areo/Tire/Front Tire/Linear Front SSC Tire/Brake model/External ==
  MBrkin : Inport
  MBrk : Outport
  wires:
  MBrkin/1 -> MBrk/1

== system In_Plane_ModelArchitecture/Chassis, Tires, and Areo/Tire/Front Tire/Linear Front SSC Tire/Brake model/MW Brake ==
  BrkPrs : Inport
  Omega : Inport  Port=2
  Brakes : Subsystem  Variant=on  VariantControlMode=label  LabelModeActiveChoice=Disk  mask{aMode=aMode}
  Gain1 : Gain  Gain=4
  Product : Product
  Tanh : Trigonometry  Operator=tanh
  Unary Minus : UnaryMinus
  MBrk : Outport
  wires:
  Product/1 -> Unary Minus/1
  Unary Minus/1 -> MBrk/1
  Gain1/1 -> Tanh/1
  Tanh/1 -> Product/2
  BrkPrs/1 -> Brakes/1(BrkPrs)
  Brakes/1(MyBrk) -> Product/1
  Omega/1 -> Brakes/2(Omega), Gain1/1

== system In_Plane_ModelArchitecture/Chassis, Tires, and Areo/Tire/Front Tire/Linear Front SSC Tire/Contact model/External ==
  Fzin : Inport
  Fz : Outport
  wires:
  Fzin/1 -> Fz/1

== system In_Plane_ModelArchitecture/Chassis, Tires, and Areo/Tire/Front Tire/Linear Front SSC Tire/Contact model/Simple spring and damper ==
  rz : Inport
  pz : Inport  Port=2
  Add4 : Sum
  Gain17 : Gain  Gain=kz
  Gain18 : Gain  Gain=cz
  Unary Minus : UnaryMinus
  contact decision : Subsystem
  Fz : Outport
  wires:
  pz/1 -> Gain17/1, contact decision/1(pos)
  Gain17/1 -> Add4/1
  Add4/1 -> contact decision/2(Fpre)
  contact decision/1(F) -> Unary Minus/1
  Gain18/1 -> Add4/2
  rz/1 -> Gain18/1
  Unary Minus/1 -> Fz/1

== system In_Plane_ModelArchitecture/Chassis, Tires, and Areo/Tire/Front Tire/Linear Front SSC Tire/Friction model/External ==
  rx : Inport
  ry : Inport  Port=2
  rz : Inport  Port=3
  Omega : Inport  Port=4
  Fxin : Inport  Port=5
  Fyin : Inport  Port=6
  Mxin : Inport  Port=7
  Myin : Inport  Port=8
  Mzin : Inport  Port=9
  Calc. part Vertical load & SideSlipAngle : Subsystem
  Mux : Mux  Inputs=3
  SlipRatio : Subsystem
  Fx : Outport
  Fy : Outport  Port=2
  Kappa : Outport  Port=3
  Alpha : Outport  Port=4
  Mx : Outport  Port=5
  My : Outport  Port=6
  Mz : Outport  Port=7
  wires:
  Omega/1 -> SlipRatio/2(Rot.Velocity)
  Calc. part Vertical load & SideSlipAngle/1(Road Vel.) -> SlipRatio/1(RoadVelocity)
  Calc. part Vertical load & SideSlipAngle/2(SideSlipAngle [rad]) -> Alpha/1
  rz/1 -> Mux/3
  ry/1 -> Mux/2
  rx/1 -> Mux/1
  Mux/1 -> Calc. part Vertical load & SideSlipAngle/1(vel.)
  Fxin/1 -> Fx/1
  Fyin/1 -> Fy/1
  SlipRatio/1(SlipRatio) -> Kappa/1
  Myin/1 -> My/1
  Mxin/1 -> Mx/1
  Mzin/1 -> Mz/1

== system In_Plane_ModelArchitecture/Chassis, Tires, and Areo/Tire/Front Tire/Linear Front SSC Tire/Friction model/Linear ==
  rx : Inport
  ry : Inport  Port=2
  rz : Inport  Port=3
  Fz : Inport  Port=4
  Omega : Inport  Port=5
  A,V,P_WhlRoll : Inport  Port=6
  Mxin : Inport  Port=7
  Myin : Inport  Port=8
  Mzin : Inport  Port=9
  Add : Sum  Inputs=--
  Bus Selector : BusSelector  OutputSignals=WhlPRoll
  Camber stiffness : Gain  Gain=kyc
  Cornering stiffness : Gain  Gain=kyl
  Divide1 : Product  Inputs=**
  Divide2 : Product  Inputs=**
  Divide3 : Product  Inputs=**
  Driving/Braking stiffness : Gain  Gain=kx
  Saturation1 : Saturate  UpperLimit=20000  LowerLimit=100  ZeroCross=off
  Slip Angle : vehdynlibtire/Dugoff Wheel 2DOF/Dugoff/Slip Angle  mask{Lrely=.001, ALPMAX=pi, ALPMIN=-pi}
      mask prompts: Lrely "Lateral relaxation length [m]:"; ALPMAX "Max slip angle [rad]:"; ALPMIN "Min slip angle [rad]:"
      settings: LibrarySourceBlock=vehdynlibtire/Fiala Wheel 2DOF/Fiala/Slip Angle
  SlipRatio : Subsystem
  Terminator : Terminator
  Terminator1 : Terminator
  Unary Minus1 : UnaryMinus
  Unary Minus3 : UnaryMinus
  Fx : Outport
  Fy : Outport  Port=2
  Kappa : Outport  Port=3
  Alpha : Outport  Port=4
  Mx : Outport  Port=5
  My : Outport  Port=6
  Mz : Outport  Port=7
  wires:
  Add/1 -> Fy/1  "Fy"
  Slip Angle/1 -> Terminator1/1
  Unary Minus3/1 -> Fx/1  "Fx"
  Divide2/1 -> Add/2  "Fyc"
  Camber stiffness/1 -> Divide2/1
  Bus Selector/1 -> Camber stiffness/1  "<WhlPRoll>"
  A,V,P_WhlRoll/1 -> Bus Selector/1
  Slip Angle/2 -> Cornering stiffness/1, Alpha/1
  Cornering stiffness/1 -> Divide3/1
  rz/1 -> Terminator/1
  Fz/1 -> Unary Minus1/1
  rx/1 -> Slip Angle/1, SlipRatio/1(RoadVelocity)
  Unary Minus1/1 -> Saturation1/1
  SlipRatio/1(SlipRatio) -> Driving/Braking stiffness/1, Kappa/1
  Omega/1 -> SlipRatio/2(Rot.Velocity)
  ry/1 -> Slip Angle/2
  Driving/Braking stiffness/1 -> Divide1/1
  Divide1/1 -> Unary Minus3/1
  Divide3/1 -> Add/1  "Fyl"
  Mxin/1 -> Mx/1
  Myin/1 -> My/1
  Mzin/1 -> Mz/1
  Saturation1/1 -> Divide2/2, Divide1/2, Divide3/2

== system In_Plane_ModelArchitecture/Chassis, Tires, and Areo/Tire/Front Tire/Linear Front SSC Tire/Simscape/Reaction Torque ==
  MWh : Inport
  Mbrk : Inport  Port=2
  External Force and Torque1 : sm_lib/Forces and Torques/External Force and Torque  EnableForceX=off  EnableForceY=off  EnableForceZ=off  EnableForce=off  ForceResolutionFrame=World  EnableTorqueX=off  EnableTorqueY=on  EnableTorqueZ=off  EnableTorque=off  TorqueResolutionFrame=AttachedFrame
  Minus1 : Sum  Inputs=--
  Simulink-PS Converter1 : nesl_utility_internal/Simulink-PS Converter  PhysicalDomain=network_engine_domain  SubClassName=ps_input  LeftPortType=input  RightPortType=output  PseudoPeriodic=off  Frequencies=[]  NoiseDistribution=none  NoiseParameters=[]  Unit=1  AffineConversion=off  FilteringAndDerivatives=provide  SimscapeFilterOrder=1  InputFilterTimeConstant=0.001  UdotUserProvided=0
  M : PMIOPort  Side=Right
  wires:
  Minus1/1 -> Simulink-PS Converter1/1
  Mbrk/1 -> Minus1/2
  MWh/1 -> Minus1/1
  connections:
  Simulink-PS Converter1/RConn1 -- External Force and Torque1/LConn1
  External Force and Torque1/RConn1 -- M/RConn1

== system In_Plane_ModelArchitecture/Chassis, Tires, and Areo/Tire/Front Tire/Linear Front SSC Tire/Simscape/Sensor ==
  PS-Simulink Converter{1..2,4..5} (4 alike) : nesl_utility_internal/PS-Simulink Converter  PhysicalDomain=network_engine_domain  SubClassName=ps_output  LeftPortType=input  RightPortType=output  PseudoPeriodic=off  Frequencies=[]  VectorFormat=1-D array  Unit=inherit  AffineConversion=off
  Transform Sensor : sm_lib/Frames and Transforms/Transform Sensor  MeasurementFrame=NonRotatingFollower  RotationSequence=XYX  SenseAngle=off  SenseAxis=off  SenseQ=off  SenseR=off  SenseRotationSequence=off  SenseOmegaX=off  SenseOmegaY=off  SenseOmegaZ=off  SenseOmega=off  SenseQDot=off  SenseRDot=off  SenseRotationSequenceDot=off  SenseAlphaX=off  SenseAlphaY=off  SenseAlphaZ=off  SenseAlpha=off  SenseQDDot=off  SenseRDDot=off  SenseX=off  SenseY=off  SenseZ=on  SenseXYZ=off  SenseRad=off  SenseAzim=off  SenseDist=off  SenseInc=off  SenseXDot=on  SenseYDot=on  SenseZDot=on  SenseXYZDot=off  SenseRadDot=off  SenseAzimDot=off  SenseDistDot=off  SenseIncDot=off  SenseXDDot=off  SenseYDDot=off  SenseZDDot=off  SenseXYZDDot=off  SenseRadDDot=off  SenseAzimDDot=off  SenseDistDDot=off  SenseIncDDot=off
  World Frame : sm_lib/Frames and Transforms/World Frame
  F : PMIOPort  Side=Left
  rx : Outport
  ry : Outport  Port=2
  rz : Outport  Port=3
  pz : Outport  Port=4
  wires:
  PS-Simulink Converter4/1 -> rz/1
  PS-Simulink Converter2/1 -> pz/1
  PS-Simulink Converter5/1 -> rx/1
  PS-Simulink Converter1/1 -> ry/1
  connections:
  Transform Sensor/LConn1 -- World Frame/RConn1
  Transform Sensor/RConn1 -- F/RConn1
  PS-Simulink Converter2/LConn1 -- Transform Sensor/RConn2
  Transform Sensor/RConn3 -- PS-Simulink Converter5/LConn1
  PS-Simulink Converter1/LConn1 -- Transform Sensor/RConn4
  PS-Simulink Converter4/LConn1 -- Transform Sensor/RConn5

== system In_Plane_ModelArchitecture/Chassis, Tires, and Areo/Tire/Front Tire/Linear Front SSC Tire/Simscape/Simscape Multibody Rim&Wheel ==
  MWh : Inport
  Fx : Inport  Port=2
  Mbrk : Inport  Port=3
  Mcr : Inport  Port=4
  Myin : Inport  Port=5
  Add_Torque : Sum  Inputs=+++
  Gain5 : Gain  Gain=RWhl
  Minus2 : Sum  Inputs=+++
  Tire_Rim_wth_transient : Subsystem
  B : PMIOPort  Side=Left
  CP : PMIOPort  Port=2  Side=Right
  omega : Outport
  omegadot : Outport  Port=2
  A,V,P_WhlRoll : Outport  Port=3
  Info_CP : Outport  Port=4
  wires:
  Tire_Rim_wth_transient/4(Info_CP) -> Info_CP/1
  Gain5/1 -> Add_Torque/2
  Tire_Rim_wth_transient/3(A,V,P_WhlRoll) -> A,V,P_WhlRoll/1
  Minus2/1 -> Add_Torque/1
  Mbrk/1 -> Add_Torque/3
  Fx/1 -> Gain5/1
  Mcr/1 -> Minus2/2
  MWh/1 -> Minus2/1
  Add_Torque/1 -> Tire_Rim_wth_transient/1(Ext.F_T)
  Tire_Rim_wth_transient/1(omega) -> omega/1
  Myin/1 -> Minus2/3
  Tire_Rim_wth_transient/2(omegadot) -> omegadot/1
  connections:
  Tire_Rim_wth_transient/LConn1 -- B/RConn1
  CP/RConn1 -- Tire_Rim_wth_transient/LConn2

== system In_Plane_ModelArchitecture/Chassis, Tires, and Areo/Tire/Front Tire/Linear Front SSC Tire/Simscape/apply forces and moments ==
  Fx : Inport
  Fy : Inport  Port=2
  Fz : Inport  Port=3
  Mxin : Inport  Port=4
  Mzin : Inport  Port=5
  External Force and Torque : sm_lib/Forces and Torques/External Force and Torque  EnableForceX=on  EnableForceY=on  EnableForceZ=on  EnableForce=off  ForceResolutionFrame=AttachedFrame  EnableTorqueX=on  EnableTorqueY=off  EnableTorqueZ=on  EnableTorque=off  TorqueResolutionFrame=AttachedFrame
  Simulink-PS Converter : nesl_utility_internal/Simulink-PS Converter  PhysicalDomain=network_engine_domain  SubClassName=ps_input  LeftPortType=input  RightPortType=output  PseudoPeriodic=off  Frequencies=[]  NoiseDistribution=none  NoiseParameters=[]  Unit=N  AffineConversion=off  FilteringAndDerivatives=zero  SimscapeFilterOrder=1  InputFilterTimeConstant=0.001  UdotUserProvided=1
  Simulink-PS Converter1 : nesl_utility_internal/Simulink-PS Converter  PhysicalDomain=network_engine_domain  SubClassName=ps_input  LeftPortType=input  RightPortType=output  PseudoPeriodic=off  Frequencies=[]  NoiseDistribution=none  NoiseParameters=[]  Unit=N  AffineConversion=off  FilteringAndDerivatives=zero  SimscapeFilterOrder=1  InputFilterTimeConstant=0.001  UdotUserProvided=1
  Simulink-PS Converter2 : nesl_utility_internal/Simulink-PS Converter  PhysicalDomain=network_engine_domain  SubClassName=ps_input  LeftPortType=input  RightPortType=output  PseudoPeriodic=off  Frequencies=[]  NoiseDistribution=none  NoiseParameters=[]  Unit=N  AffineConversion=off  FilteringAndDerivatives=zero  SimscapeFilterOrder=1  InputFilterTimeConstant=0.001  UdotUserProvided=1
  Simulink-PS Converter3 : nesl_utility_internal/Simulink-PS Converter  PhysicalDomain=network_engine_domain  SubClassName=ps_input  LeftPortType=input  RightPortType=output  PseudoPeriodic=off  Frequencies=[]  NoiseDistribution=none  NoiseParameters=[]  Unit=N*m  AffineConversion=off  FilteringAndDerivatives=zero  SimscapeFilterOrder=1  InputFilterTimeConstant=0.001  UdotUserProvided=1
  Simulink-PS Converter4 : nesl_utility_internal/Simulink-PS Converter  PhysicalDomain=network_engine_domain  SubClassName=ps_input  LeftPortType=input  RightPortType=output  PseudoPeriodic=off  Frequencies=[]  NoiseDistribution=none  NoiseParameters=[]  Unit=N*m  AffineConversion=off  FilteringAndDerivatives=zero  SimscapeFilterOrder=1  InputFilterTimeConstant=0.001  UdotUserProvided=1
  CP : PMIOPort  Side=Right
  wires:
  Fx/1 -> Simulink-PS Converter/1
  Fz/1 -> Simulink-PS Converter2/1
  Fy/1 -> Simulink-PS Converter1/1
  Mxin/1 -> Simulink-PS Converter3/1
  Mzin/1 -> Simulink-PS Converter4/1
  connections:
  External Force and Torque/LConn3 -- Simulink-PS Converter2/RConn1
  External Force and Torque/LConn1 -- Simulink-PS Converter/RConn1
  External Force and Torque/RConn1 -- CP/RConn1
  Simulink-PS Converter1/RConn1 -- External Force and Torque/LConn2
  External Force and Torque/LConn4 -- Simulink-PS Converter3/RConn1
  External Force and Torque/LConn5 -- Simulink-PS Converter4/RConn1

== system In_Plane_ModelArchitecture/Chassis, Tires, and Areo/Tire/Rear Tire/Linear Rear SSC Tire/Brake model/External ==
  MBrkin : Inport
  MBrk : Outport
  wires:
  MBrkin/1 -> MBrk/1
